simulink library "halout"  (R2024a)
settings: Solver=VariableStepAuto  StartTime=0.0  StopTime=10.0  RelTol=1e-3
undefined symbols (not defined in the file): KHAL_CAN3TxReq_flg, KHAL_CAN_MCU_R1TxReq_flg, TRUE
libraries: FVT_lib x20, simulink x1
settings Model: Creator=13168  LastModifiedBy=FVT22063
settings SolverCC: AlgebraicLoopSolver=TrustRegion
settings DataIOCC: SaveFormat=Array  SignalLoggingSaveFormat=ModelDataLogs  ReturnWorkspaceOutputs=off
settings OptimizationCC: BlockReduction=off  BooleanDataType=off
settings DebuggingCC: SaveWithParameterizedLinksMsg=none  UnderspecifiedInitializationDetection=Classic  MergeDetectMultiDrivingBlocksExec=none  SignalResolutionControl=TryResolveAllWithWarning  UnconnectedInputMsg=warning  UnconnectedOutputMsg=warning  UnconnectedLineMsg=warning
settings HardwareCC: TargetUnknown=on
settings ModelReferenceCC: EnableRefExpFcnMdlSchedulingChecks=on  PropagateSignalLabelsOutOfModel=off
settings RTWCC: GPUComputeCapability=3.5  DLArmComputeVersion=19.05
settings ConfigComp: CovMetricSettings=dw  CovSaveCumulativeToWorkspaceVar=on  CovSaveSingleToWorkspaceVar=on

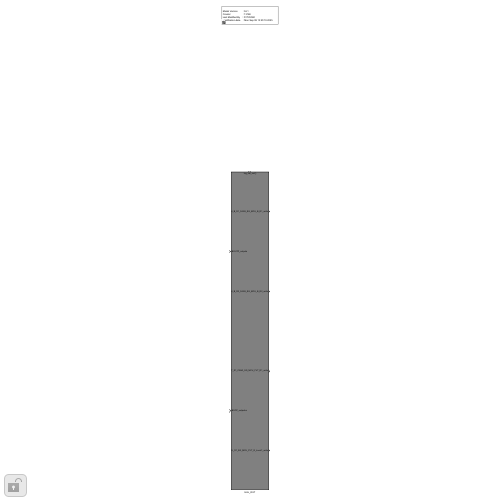
[thumbnail: Simulink's stored preview of the top-level diagram]
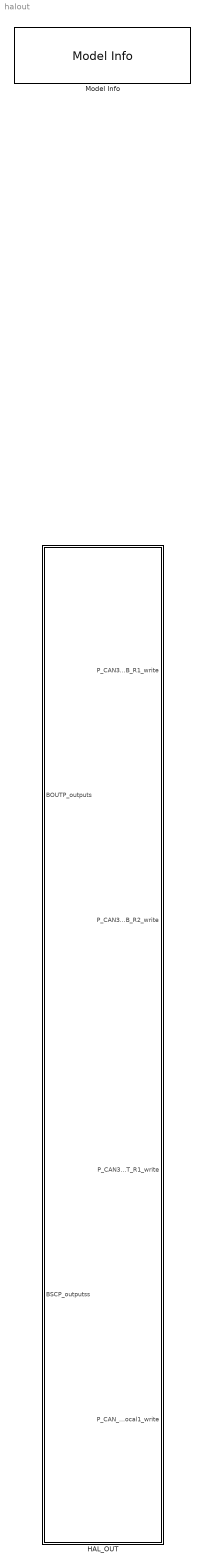
== system halout ==
  HAL_OUT : Subsystem
      settings: RTWSystemCode=Nonreusable function  RTWFcnNameOpts=Use subsystem name  RTWFileNameOpts=Use subsystem name
  Model Info : simulink/Model-Wide Utilities/Model Info  Frame=on  DisplayStringWithTags=|  HorizontalTextAlignment=Left  LeftAlignmentValue=0.02
      | Model Version        : %<ModelVersion>
      | Creator                   : %<Creator>
      | Last Modified By    : %<LastModifiedBy>
      | Modification date    : %<LastModificationDate>

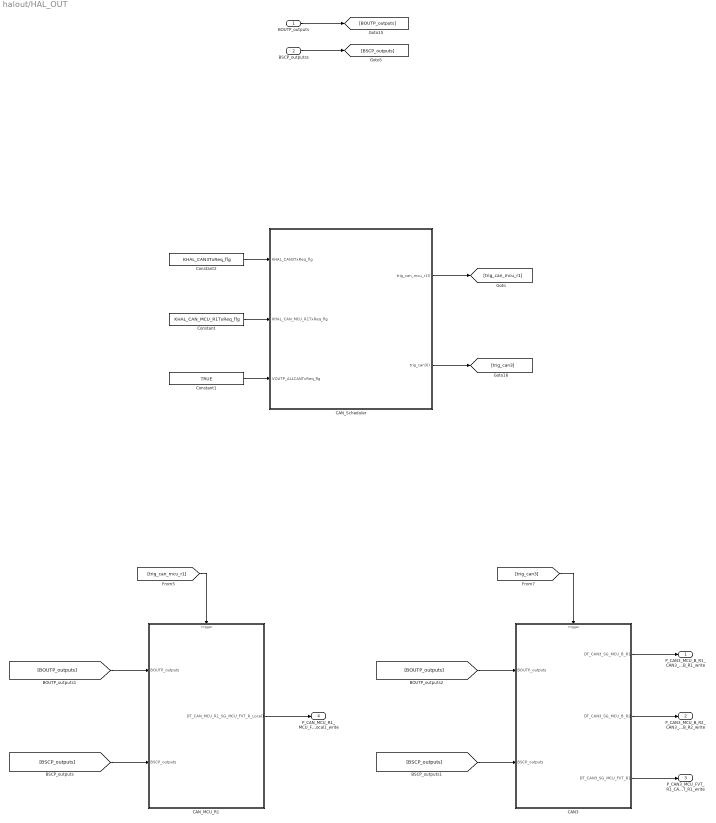
== system halout/HAL_OUT ==
  BOUTP_outputs : Inport  OutDataTypeStr=Bus: BOUTP_outputs
  BSCP_outputss : Inport  Port=2  OutDataTypeStr=Bus:BSCP_outputs
  CAN3 : Subsystem  TreatAsAtomicUnit=on
  CAN_MCU_R1 : Subsystem  TreatAsAtomicUnit=on
  CAN_Scheduler : Stateflow chart  TreatAsAtomicUnit=on
      settings: PortSchema="{\"entries\":[{\"content\":{\"sides\":[{\"content\":{\"connectorIds\":[\"In1\",\"In3\",\"In2\"]},\"type\":\"ConnectorPlacement.EquallySpacedRectSide\",\"uuid\":\"eca17bd2-3cd0-45cb-a786-10f6e0edb75c\"},{\"content\":{\"connectorIds\":[\"Out1\",\"Out2\"],\"side\":\"RIGHT\"},\"type\":\"ConnectorPlacement.EquallySpacedRectSide\",\"uuid\":\"6e53f934-0f1a-471e-8062-0040e0751220\"},{\"content\":{\"side\":\"TOP\"},\"type\":\"ConnectorPlacement.EquallySpacedRectSide\",\"uuid\":\"8d6d34ea-7fb8-416e-91ba-08d9a797d464\"}]},\"type\":\"ConnectorPlacement.EquallySpacedConnector\",\"uuid\":\"7b75ce71-1842-4580-bcde-4badbb5525c1\"}],\"packageUris\":[\"http://schema.mathworks.com/mf0/Connector/R2020b\"],\"version\":\"1.0\"}"
  Constant : Constant  Value=KHAL_CAN_MCU_R1TxReq_flg
  Constant1 : Constant  Value=TRUE  OutDataTypeStr=boolean
  Constant2 : Constant  Value=KHAL_CAN3TxReq_flg
  P_CAN3_MCU_B_R1_CAN3_SG_MCU_B_R1_write : Outport  OutDataTypeStr=Bus: DT_CAN3_SG_MCU_B_R1
  P_CAN3_MCU_B_R2_CAN3_SG_MCU_B_R2_write : Outport  Port=2  OutDataTypeStr=Bus: DT_CAN3_SG_MCU_B_R2
  P_CAN3_MCU_FVT_R1_CAN3_SG_MCU_FVT_R1_write : Outport  Port=3  OutDataTypeStr=Bus: DT_CAN3_SG_MCU_FVT_R1
  P_CAN_MCU_R1_MCU_FVT_R_Local1_CAN_MCU_R1_SG_MCU_FVT_R_Local1_write : Outport  Port=4  OutDataTypeStr=Bus: DT_CAN_MCU_R1_SG_MCU_FVT_R_Local1
  wires:
  BSCP_outputss/1 -> [BSCP_outputs]
  BOUTP_outputs/1 -> [BOUTP_outputs]
  Constant/1 -> CAN_Scheduler/3(KHAL_CAN_MCU_R1TxReq_flg)
  Constant2/1 -> CAN_Scheduler/1(KHAL_CAN3TxReq_flg)
  Constant1/1 -> CAN_Scheduler/2(VOUTP_ALLCANTxReq_flg)
  CAN_Scheduler/2(trig_can3()) -> [trig_can3]
  CAN_Scheduler/1(trig_can_mcu_r1()) -> [trig_can_mcu_r1]
  [trig_can3] -> CAN3/Trigger
  [trig_can_mcu_r1] -> CAN_MCU_R1/Trigger
  [BOUTP_outputs] -> CAN3/1(BOUTP_outputs)
  CAN3/2(DT_CAN3_SG_MCU_B_R2) -> P_CAN3_MCU_B_R2_CAN3_SG_MCU_B_R2_write/1
  [BSCP_outputs] -> CAN_MCU_R1/2(BSCP_outputs)
  [BOUTP_outputs] -> CAN_MCU_R1/1(BOUTP_outputs)
  CAN3/1(DT_CAN3_SG_MCU_B_R1) -> P_CAN3_MCU_B_R1_CAN3_SG_MCU_B_R1_write/1
  CAN_MCU_R1/1(DT_CAN_MCU_R1_SG_MCU_FVT_R_Local1) -> P_CAN_MCU_R1_MCU_FVT_R_Local1_CAN_MCU_R1_SG_MCU_FVT_R_Local1_write/1
  [BSCP_outputs] -> CAN3/2(BSCP_outputs)
  CAN3/3(DT_CAN3_SG_MCU_FVT_R1) -> P_CAN3_MCU_FVT_R1_CAN3_SG_MCU_FVT_R1_write/1

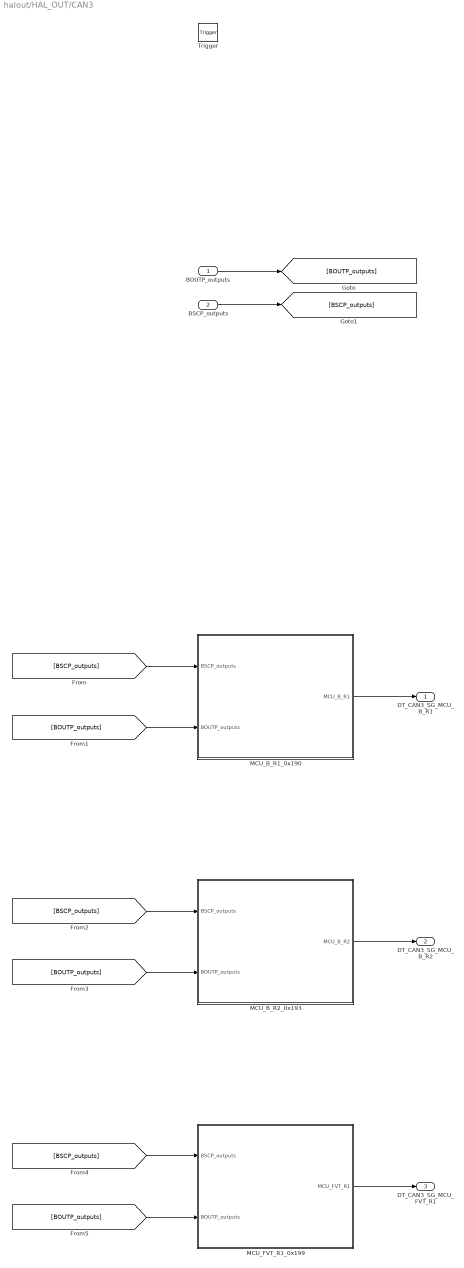
== system halout/HAL_OUT/CAN3 ==
  BOUTP_outputs : Inport  OutDataTypeStr=Bus: BOUTP_outputs
  BSCP_outputs : Inport  Port=2  OutDataTypeStr=Bus: BSCP_outputs
  Trigger : TriggerPort  TriggerType=function-call  VariantControl=(inherit)
  MCU_B_R1_0x190 : Subsystem
  MCU_B_R2_0x193 : Subsystem
  MCU_FVT_R1_0x199 : Subsystem
  DT_CAN3_SG_MCU_B_R1 : Outport  OutDataTypeStr=Bus: DT_CAN3_SG_MCU_B_R1
  DT_CAN3_SG_MCU_B_R2 : Outport  Port=2  OutDataTypeStr=Bus: DT_CAN3_SG_MCU_B_R2
  DT_CAN3_SG_MCU_FVT_R1 : Outport  Port=3  OutDataTypeStr=Bus: DT_CAN3_SG_MCU_FVT_R1
  wires:
  BOUTP_outputs/1 -> [BOUTP_outputs]
  BSCP_outputs/1 -> [BSCP_outputs]
  [BSCP_outputs] -> MCU_B_R1_0x190/1(BSCP_outputs)
  [BOUTP_outputs] -> MCU_B_R1_0x190/2(BOUTP_outputs)
  MCU_B_R1_0x190/1(MCU_B_R1) -> DT_CAN3_SG_MCU_B_R1/1
  [BSCP_outputs] -> MCU_B_R2_0x193/1(BSCP_outputs)
  [BOUTP_outputs] -> MCU_B_R2_0x193/2(BOUTP_outputs)
  MCU_B_R2_0x193/1(MCU_B_R2) -> DT_CAN3_SG_MCU_B_R2/1
  [BSCP_outputs] -> MCU_FVT_R1_0x199/1(BSCP_outputs)
  [BOUTP_outputs] -> MCU_FVT_R1_0x199/2(BOUTP_outputs)
  MCU_FVT_R1_0x199/1(MCU_FVT_R1) -> DT_CAN3_SG_MCU_FVT_R1/1

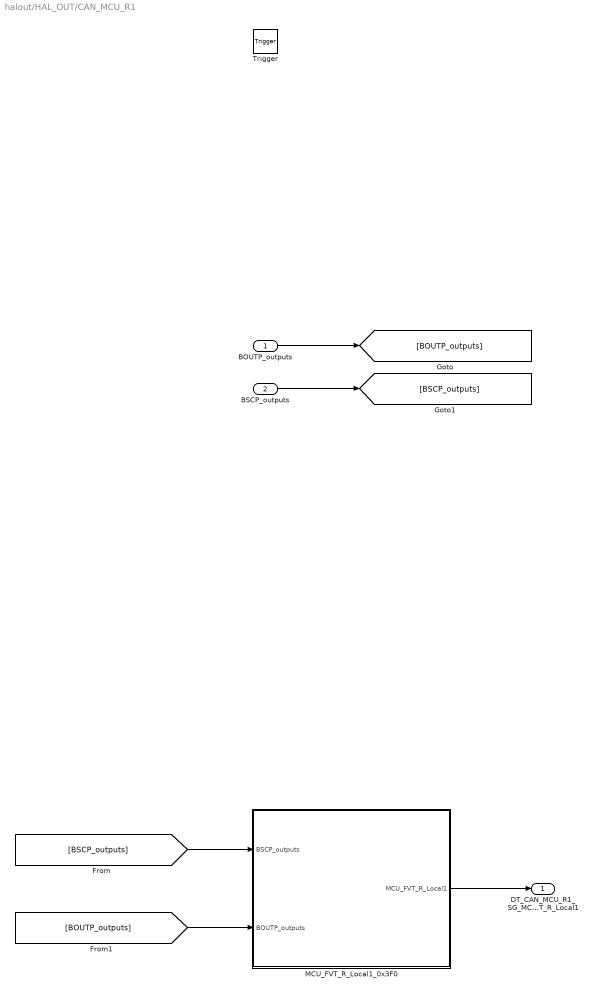
== system halout/HAL_OUT/CAN_MCU_R1 ==
  BOUTP_outputs : Inport  OutDataTypeStr=Bus: BOUTP_outputs
  BSCP_outputs : Inport  Port=2  OutDataTypeStr=Bus: BSCP_outputs
  Trigger : TriggerPort  TriggerType=function-call  VariantControl=(inherit)
  MCU_FVT_R_Local1_0x3F0 : Subsystem
  DT_CAN_MCU_R1_SG_MCU_FVT_R_Local1 : Outport  OutDataTypeStr=Bus: DT_CAN_MCU_R1_SG_MCU_FVT_R_Local1
  wires:
  BOUTP_outputs/1 -> [BOUTP_outputs]
  BSCP_outputs/1 -> [BSCP_outputs]
  [BSCP_outputs] -> MCU_FVT_R_Local1_0x3F0/1(BSCP_outputs)
  [BOUTP_outputs] -> MCU_FVT_R_Local1_0x3F0/2(BOUTP_outputs)
  MCU_FVT_R_Local1_0x3F0/1(MCU_FVT_R_Local1) -> DT_CAN_MCU_R1_SG_MCU_FVT_R_Local1/1

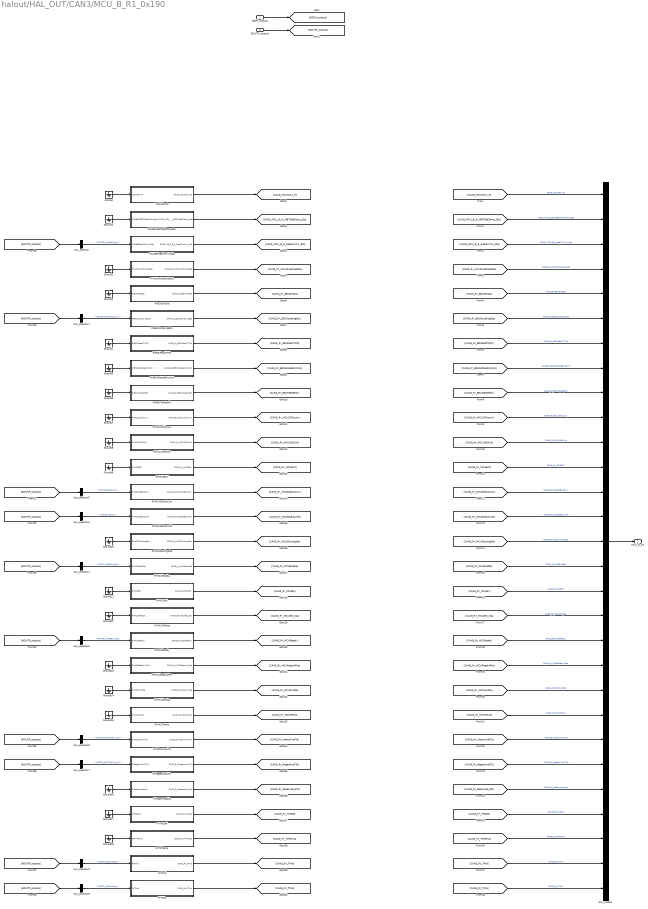
== system halout/HAL_OUT/CAN3/MCU_B_R1_0x190 ==
  BSCP_outputs : Inport  OutDataTypeStr=Bus: BSCP_outputs
  BOUTP_outputs : Inport  Port=2  OutDataTypeStr=Bus: BOUTP_outputs
  Ground{,1..18} (19 alike) : Ground
  MCUBRIGBTDdeTempSta : Subsystem
  MCUBRRealPwrKwSta : Subsystem
  MCUWarnR : Subsystem
  RrActvDmpDisabSta : Subsystem
  RrEDUDrtSta : Subsystem
  RrEDUOpratingSta : Subsystem
  RrEDURealTMTq : Subsystem
  RrEDURotateDirction : Subsystem
  RrEDUTqReqFbk : Subsystem
  RrMCU1Chksum : Subsystem
  RrMCU1RolCnt : Subsystem
  RrMCUBAT : Subsystem
  RrMCUDCBusCurr : Subsystem
  RrMCUDCBusVolt : Subsystem
  RrMCUDischrgSta : Subsystem
  RrMCUEnaSta : Subsystem
  RrMCUErr : Subsystem
  RrMCUIGNsta : Subsystem
  RrMCUReady : Subsystem
  RrMCUReady4Pre : Subsystem
  RrMCUSysSta : Subsystem
  RrMCUTemp : Subsystem
  RrMotorAvailTq : Subsystem
  RrRegenAvailTq : Subsystem
  RrReservedbits : Subsystem
  RrTMSpd : Subsystem
  RrTMTemp : Subsystem
  RrTMid : Subsystem
  RrTMiq : Subsystem
  bus_creator : BusCreator  Inputs=29  OutDataTypeStr=Bus: DT_CAN3_SG_MCU_B_R1  NonVirtualBus=on
  bus_selector : BusSelector  OutputSignals=VOUTP_PwrEleAct_W
  bus_selector1 : BusSelector  OutputSignals=VOUTP_MotMod_enum
  bus_selector2 : BusSelector  OutputSignals=VOUTP_BusCurr_A
  bus_selector3 : BusSelector  OutputSignals=VOUTP_uDC_V
  bus_selector4 : BusSelector  OutputSignals=VOUTP_MCUEna_flg
  bus_selector5 : BusSelector  OutputSignals=VOUTP_TMReady_flg
  bus_selector6 : BusSelector  OutputSignals=VOUTP_tqTMTqMax_Nm
  bus_selector7 : BusSelector  OutputSignals=VOUTP_tqTMTqMin_Nm
  bus_selector8 : BusSelector  OutputSignals=VOUTP_iDCurrAct_A
  bus_selector9 : BusSelector  OutputSignals=VOUTP_iQCurrAct_A
  MCU_B_R1 : Outport
  wires:
  BSCP_outputs/1 -> [BSCP_outputs]
  BOUTP_outputs/1 -> [BOUTP_outputs]
  [CAN3_MCUWarn_R] -> bus_creator/1  "CAN3_MCUWarn_R"
  [CAN3_MCU_B_R_IGBTDdeTemp_Sta] -> bus_creator/2  "CAN3_MCU_B_R_IGBTDdeTemp_Sta"
  [CAN3_MCU_B_R_RealPwrKw_Sta] -> bus_creator/3  "CAN3_MCU_B_R_RealPwrKw_Sta"
  [CAN3_Rr_ActvDmpDisabSta] -> bus_creator/4  "CAN3_Rr_ActvDmpDisabSta"
  [CAN3_Rr_EDUDrtSta] -> bus_creator/5  "CAN3_Rr_EDUDrtSta"
  [CAN3_Rr_EDUOpratingSta] -> bus_creator/6  "CAN3_Rr_EDUOpratingSta"
  [CAN3_Rr_EDURealTMTq] -> bus_creator/7  "CAN3_Rr_EDURealTMTq"
  [CAN3_Rr_EDURotateDirction] -> bus_creator/8  "CAN3_Rr_EDURotateDirction"
  [CAN3_Rr_EDUTqReqFbk] -> bus_creator/9  "CAN3_Rr_EDUTqReqFbk"
  [CAN3_Rr_MCU1Chksum] -> bus_creator/10  "CAN3_Rr_MCU1Chksum"
  [CAN3_Rr_MCU1RolCnt] -> bus_creator/11  "CAN3_Rr_MCU1RolCnt"
  [CAN3_Rr_MCUBAT] -> bus_creator/12  "CAN3_Rr_MCUBAT"
  [CAN3_Rr_MCUDCBusCurr] -> bus_creator/13  "CAN3_Rr_MCUDCBusCurr"
  [CAN3_Rr_MCUDCBusVolt] -> bus_creator/14  "CAN3_Rr_MCUDCBusVolt"
  [CAN3_Rr_MCUDischrgSta] -> bus_creator/15  "CAN3_Rr_MCUDischrgSta"
  [CAN3_Rr_MCUEnaSta] -> bus_creator/16  "CAN3_Rr_MCUEnaSta"
  [CAN3_Rr_MCUErr] -> bus_creator/17  "CAN3_Rr_MCUErr"
  [CAN3_Rr_MCUIGN_sta] -> bus_creator/18  "CAN3_Rr_MCUIGN_sta"
  [CAN3_Rr_MCUReady] -> bus_creator/19  "CAN3_Rr_MCUReady"
  [CAN3_Rr_MCUReady4Pre] -> bus_creator/20  "CAN3_Rr_MCUReady4Pre"
  [CAN3_Rr_MCUSysSta] -> bus_creator/21  "CAN3_Rr_MCUSysSta"
  [CAN3_Rr_MCUTemp] -> bus_creator/22  "CAN3_Rr_MCUTemp"
  [CAN3_Rr_MotorAvailTq] -> bus_creator/23  "CAN3_Rr_MotorAvailTq"
  [CAN3_Rr_RegenAvailTq] -> bus_creator/24  "CAN3_Rr_RegenAvailTq"
  [CAN3_Rr_Reserved_bits] -> bus_creator/25  "CAN3_Rr_Reserved_bits"
  [CAN3_Rr_TMSpd] -> bus_creator/26  "CAN3_Rr_TMSpd"
  [CAN3_Rr_TMTemp] -> bus_creator/27  "CAN3_Rr_TMTemp"
  [CAN3_Rr_TMid] -> bus_creator/28  "CAN3_Rr_TMid"
  [CAN3_Rr_TMiq] -> bus_creator/29  "CAN3_Rr_TMiq"
  bus_creator/1 -> MCU_B_R1/1
  MCUWarnR/1(CAN3_MCUWarn_R) -> [CAN3_MCUWarn_R]
  MCUBRIGBTDdeTempSta/1(CAN3_MCU_B_R_IGBTDdeTemp_Sta) -> [CAN3_MCU_B_R_IGBTDdeTemp_Sta]
  MCUBRRealPwrKwSta/1(CAN3_MCU_B_R_RealPwrKw_Sta) -> [CAN3_MCU_B_R_RealPwrKw_Sta]
  RrActvDmpDisabSta/1(CAN3_Rr_ActvDmpDisabSta) -> [CAN3_Rr_ActvDmpDisabSta]
  RrEDUDrtSta/1(CAN3_Rr_EDUDrtSta) -> [CAN3_Rr_EDUDrtSta]
  RrEDUOpratingSta/1(CAN3_Rr_EDUOpratingSta) -> [CAN3_Rr_EDUOpratingSta]
  RrEDURealTMTq/1(CAN3_Rr_EDURealTMTq) -> [CAN3_Rr_EDURealTMTq]
  RrEDURotateDirction/1(CAN3_Rr_EDURotateDirction) -> [CAN3_Rr_EDURotateDirction]
  RrEDUTqReqFbk/1(CAN3_Rr_EDUTqReqFbk) -> [CAN3_Rr_EDUTqReqFbk]
  RrMCU1Chksum/1(CAN3_Rr_MCU1Chksum) -> [CAN3_Rr_MCU1Chksum]
  RrMCU1RolCnt/1(CAN3_Rr_MCU1RolCnt) -> [CAN3_Rr_MCU1RolCnt]
  RrMCUBAT/1(CAN3_Rr_MCUBAT) -> [CAN3_Rr_MCUBAT]
  RrMCUDCBusCurr/1(CAN3_Rr_MCUDCBusCurr) -> [CAN3_Rr_MCUDCBusCurr]
  RrMCUDCBusVolt/1(CAN3_Rr_MCUDCBusVolt) -> [CAN3_Rr_MCUDCBusVolt]
  RrMCUDischrgSta/1(CAN3_Rr_MCUDischrgSta) -> [CAN3_Rr_MCUDischrgSta]
  RrMCUEnaSta/1(CAN3_Rr_MCUEnaSta) -> [CAN3_Rr_MCUEnaSta]
  RrMCUErr/1(CAN3_Rr_MCUErr) -> [CAN3_Rr_MCUErr]
  RrMCUIGNsta/1(CAN3_Rr_MCUIGN_sta) -> [CAN3_Rr_MCUIGN_sta]
  RrMCUReady/1(CAN3_Rr_MCUReady) -> [CAN3_Rr_MCUReady]
  RrMCUReady4Pre/1(CAN3_Rr_MCUReady4Pre) -> [CAN3_Rr_MCUReady4Pre]
  RrMCUSysSta/1(CAN3_Rr_MCUSysSta) -> [CAN3_Rr_MCUSysSta]
  RrMCUTemp/1(CAN3_Rr_MCUTemp) -> [CAN3_Rr_MCUTemp]
  RrMotorAvailTq/1(CAN3_Rr_MotorAvailTq) -> [CAN3_Rr_MotorAvailTq]
  RrRegenAvailTq/1(CAN3_Rr_RegenAvailTq) -> [CAN3_Rr_RegenAvailTq]
  RrReservedbits/1(CAN3_Rr_Reserved_bits) -> [CAN3_Rr_Reserved_bits]
  RrTMSpd/1(CAN3_Rr_TMSpd) -> [CAN3_Rr_TMSpd]
  RrTMTemp/1(CAN3_Rr_TMTemp) -> [CAN3_Rr_TMTemp]
  RrTMid/1(CAN3_Rr_TMid) -> [CAN3_Rr_TMid]
  RrTMiq/1(CAN3_Rr_TMiq) -> [CAN3_Rr_TMiq]
  Ground/1 -> MCUWarnR/1(MCUWarnR)
  Ground1/1 -> MCUBRIGBTDdeTempSta/1(MCUBRIGBTDdeTempSta)
  bus_selector/1 -> MCUBRRealPwrKwSta/1(MCUBRRealPwrKwSta)  "<VOUTP_PwrEleAct_W>"
  [BOUTP_outputs] -> bus_selector/1
  Ground2/1 -> RrActvDmpDisabSta/1(RrActvDmpDisabSta)
  Ground3/1 -> RrEDUDrtSta/1(RrEDUDrtSta)
  bus_selector1/1 -> RrEDUOpratingSta/1(RrEDUOpratingSta)  "<VOUTP_MotMod_enum>"
  [BOUTP_outputs] -> bus_selector1/1
  Ground4/1 -> RrEDURealTMTq/1(RrEDURealTMTq)
  Ground5/1 -> RrEDURotateDirction/1(RrEDURotateDirction)
  Ground6/1 -> RrEDUTqReqFbk/1(RrEDUTqReqFbk)
  Ground7/1 -> RrMCU1Chksum/1(RrMCU1Chksum)
  Ground8/1 -> RrMCU1RolCnt/1(RrMCU1RolCnt)
  Ground9/1 -> RrMCUBAT/1(RrMCUBAT)
  bus_selector2/1 -> RrMCUDCBusCurr/1(RrMCUDCBusCurr)  "<VOUTP_BusCurr_A>"
  [BOUTP_outputs] -> bus_selector2/1
  bus_selector3/1 -> RrMCUDCBusVolt/1(RrMCUDCBusVolt)  "<VOUTP_uDC_V>"
  [BOUTP_outputs] -> bus_selector3/1
  Ground10/1 -> RrMCUDischrgSta/1(RrMCUDischrgSta)
  bus_selector4/1 -> RrMCUEnaSta/1(RrMCUEnaSta)  "<VOUTP_MCUEna_flg>"
  [BOUTP_outputs] -> bus_selector4/1
  Ground11/1 -> RrMCUErr/1(RrMCUErr)
  Ground12/1 -> RrMCUIGNsta/1(RrMCUIGNsta)
  bus_selector5/1 -> RrMCUReady/1(RrMCUReady)  "<VOUTP_TMReady_flg>"
  [BOUTP_outputs] -> bus_selector5/1
  Ground13/1 -> RrMCUReady4Pre/1(RrMCUReady4Pre)
  Ground14/1 -> RrMCUSysSta/1(RrMCUSysSta)
  Ground15/1 -> RrMCUTemp/1(RrMCUTemp)
  bus_selector6/1 -> RrMotorAvailTq/1(RrMotorAvailTq)  "<VOUTP_tqTMTqMax_Nm>"
  [BOUTP_outputs] -> bus_selector6/1
  bus_selector7/1 -> RrRegenAvailTq/1(RrRegenAvailTq)  "<VOUTP_tqTMTqMin_Nm>"
  [BOUTP_outputs] -> bus_selector7/1
  Ground16/1 -> RrReservedbits/1(RrReservedbits)
  Ground17/1 -> RrTMSpd/1(RrTMSpd)
  Ground18/1 -> RrTMTemp/1(RrTMTemp)
  bus_selector8/1 -> RrTMid/1(RrTMid)  "<VOUTP_iDCurrAct_A>"
  [BOUTP_outputs] -> bus_selector8/1
  bus_selector9/1 -> RrTMiq/1(RrTMiq)  "<VOUTP_iQCurrAct_A>"
  [BOUTP_outputs] -> bus_selector9/1

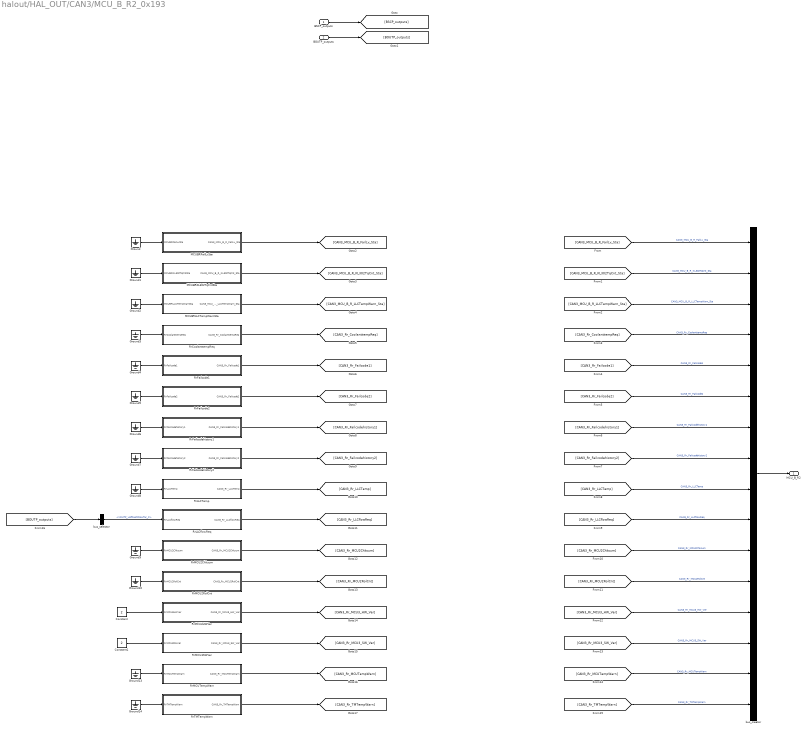
== system halout/HAL_OUT/CAN3/MCU_B_R2_0x193 ==
  BSCP_outputs : Inport  OutDataTypeStr=Bus: BSCP_outputs
  BOUTP_outputs : Inport  Port=2  OutDataTypeStr=Bus: BOUTP_outputs
  Constant : Constant  Value=2
  Constant1 : Constant  Value=2
  Ground{,1..10,13..14} (13 alike) : Ground
  MCUBRFailLvSta : Subsystem
  MCUBRKL302TqCntSta : Subsystem
  MCUBRLLCTempWarnSta : Subsystem
  RrCoolanttempReq : Subsystem
  RrFailcode1 : Subsystem
  RrFailcode2 : Subsystem
  RrFailcodehistory1 : Subsystem
  RrFailcodehistory2 : Subsystem
  RrLLCTemp : Subsystem
  RrLLCflowReq : Subsystem
  RrMCU2Chksum : Subsystem
  RrMCU2RolCnt : Subsystem
  RrMCU3HWVer : Subsystem
  RrMCU3SWVer : Subsystem
  RrMCUTempWarn : Subsystem
  RrTMTempWarn : Subsystem
  bus_creator : BusCreator  Inputs=16  OutDataTypeStr=Bus: DT_CAN3_SG_MCU_B_R2  NonVirtualBus=on
  bus_selector : BusSelector  OutputSignals=VOUTP_volfCooltFlowTar_C
  MCU_B_R2 : Outport
  wires:
  BSCP_outputs/1 -> [BSCP_outputs]
  BOUTP_outputs/1 -> [BOUTP_outputs]
  [CAN3_MCU_B_R_FailLv_Sta] -> bus_creator/1  "CAN3_MCU_B_R_FailLv_Sta"
  [CAN3_MCU_B_R_KL302TqCnt_Sta] -> bus_creator/2  "CAN3_MCU_B_R_KL302TqCnt_Sta"
  [CAN3_MCU_B_R_LLCTempWarn_Sta] -> bus_creator/3  "CAN3_MCU_B_R_LLCTempWarn_Sta"
  [CAN3_Rr_CoolanttempReq] -> bus_creator/4  "CAN3_Rr_CoolanttempReq"
  [CAN3_Rr_Failcode1] -> bus_creator/5  "CAN3_Rr_Failcode1"
  [CAN3_Rr_Failcode2] -> bus_creator/6  "CAN3_Rr_Failcode2"
  [CAN3_Rr_Failcodehistory1] -> bus_creator/7  "CAN3_Rr_Failcodehistory1"
  [CAN3_Rr_Failcodehistory2] -> bus_creator/8  "CAN3_Rr_Failcodehistory2"
  [CAN3_Rr_LLCTemp] -> bus_creator/9  "CAN3_Rr_LLCTemp"
  [CAN3_Rr_LLCflowReq] -> bus_creator/10  "CAN3_Rr_LLCflowReq"
  [CAN3_Rr_MCU2Chksum] -> bus_creator/11  "CAN3_Rr_MCU2Chksum"
  [CAN3_Rr_MCU2RolCnt] -> bus_creator/12  "CAN3_Rr_MCU2RolCnt"
  [CAN3_Rr_MCU3_HW_Ver] -> bus_creator/13  "CAN3_Rr_MCU3_HW_Ver"
  [CAN3_Rr_MCU3_SW_Ver] -> bus_creator/14  "CAN3_Rr_MCU3_SW_Ver"
  [CAN3_Rr_MCUTempWarn] -> bus_creator/15  "CAN3_Rr_MCUTempWarn"
  [CAN3_Rr_TMTempWarn] -> bus_creator/16  "CAN3_Rr_TMTempWarn"
  bus_creator/1 -> MCU_B_R2/1
  MCUBRFailLvSta/1(CAN3_MCU_B_R_FailLv_Sta) -> [CAN3_MCU_B_R_FailLv_Sta]
  MCUBRKL302TqCntSta/1(CAN3_MCU_B_R_KL302TqCnt_Sta) -> [CAN3_MCU_B_R_KL302TqCnt_Sta]
  MCUBRLLCTempWarnSta/1(CAN3_MCU_B_R_LLCTempWarn_Sta) -> [CAN3_MCU_B_R_LLCTempWarn_Sta]
  RrCoolanttempReq/1(CAN3_Rr_CoolanttempReq) -> [CAN3_Rr_CoolanttempReq]
  RrFailcode1/1(CAN3_Rr_Failcode1) -> [CAN3_Rr_Failcode1]
  RrFailcode2/1(CAN3_Rr_Failcode2) -> [CAN3_Rr_Failcode2]
  RrFailcodehistory1/1(CAN3_Rr_Failcodehistory1) -> [CAN3_Rr_Failcodehistory1]
  RrFailcodehistory2/1(CAN3_Rr_Failcodehistory2) -> [CAN3_Rr_Failcodehistory2]
  RrLLCTemp/1(CAN3_Rr_LLCTemp) -> [CAN3_Rr_LLCTemp]
  RrLLCflowReq/1(CAN3_Rr_LLCflowReq) -> [CAN3_Rr_LLCflowReq]
  RrMCU2Chksum/1(CAN3_Rr_MCU2Chksum) -> [CAN3_Rr_MCU2Chksum]
  RrMCU2RolCnt/1(CAN3_Rr_MCU2RolCnt) -> [CAN3_Rr_MCU2RolCnt]
  RrMCU3HWVer/1(CAN3_Rr_MCU3_HW_Ver) -> [CAN3_Rr_MCU3_HW_Ver]
  RrMCU3SWVer/1(CAN3_Rr_MCU3_SW_Ver) -> [CAN3_Rr_MCU3_SW_Ver]
  RrMCUTempWarn/1(CAN3_Rr_MCUTempWarn) -> [CAN3_Rr_MCUTempWarn]
  RrTMTempWarn/1(CAN3_Rr_TMTempWarn) -> [CAN3_Rr_TMTempWarn]
  Ground/1 -> MCUBRFailLvSta/1(MCUBRFailLvSta)
  Ground1/1 -> MCUBRKL302TqCntSta/1(MCUBRKL302TqCntSta)
  Ground2/1 -> MCUBRLLCTempWarnSta/1(MCUBRLLCTempWarnSta)
  Ground3/1 -> RrCoolanttempReq/1(RrCoolanttempReq)
  Ground4/1 -> RrFailcode1/1(RrFailcode1)
  Ground5/1 -> RrFailcode2/1(RrFailcode2)
  Ground6/1 -> RrFailcodehistory1/1(RrFailcodehistory1)
  Ground7/1 -> RrFailcodehistory2/1(RrFailcodehistory2)
  Ground8/1 -> RrLLCTemp/1(RrLLCTemp)
  bus_selector/1 -> RrLLCflowReq/1(RrLLCflowReq)  "<VOUTP_volfCooltFlowTar_C>"
  [BOUTP_outputs] -> bus_selector/1
  Ground9/1 -> RrMCU2Chksum/1(RrMCU2Chksum)
  Ground10/1 -> RrMCU2RolCnt/1(RrMCU2RolCnt)
  Constant/1 -> RrMCU3HWVer/1(RrMCU3HWVer)
  Constant1/1 -> RrMCU3SWVer/1(RrMCU3SWVer)
  Ground13/1 -> RrMCUTempWarn/1(RrMCUTempWarn)
  Ground14/1 -> RrTMTempWarn/1(RrTMTempWarn)

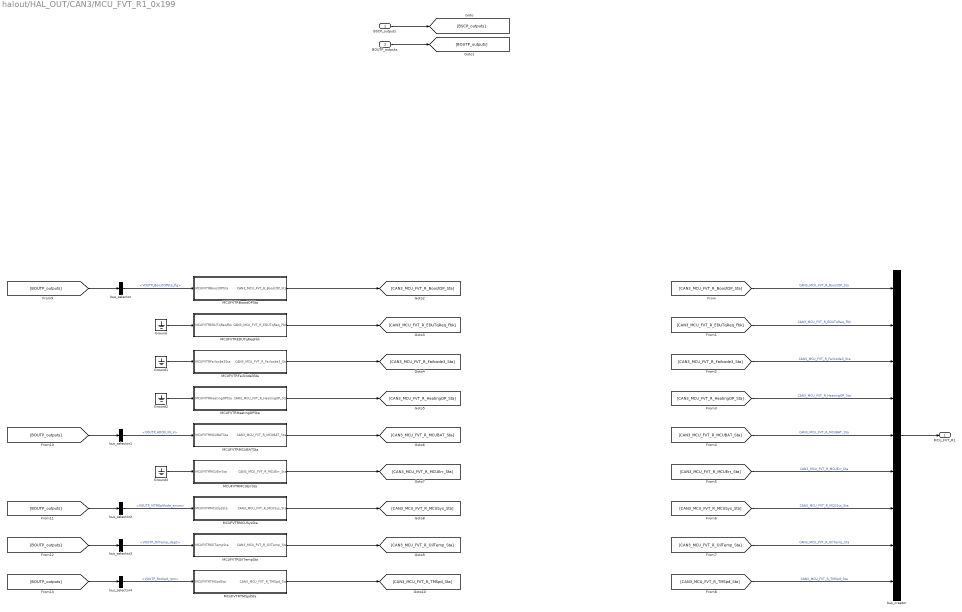
== system halout/HAL_OUT/CAN3/MCU_FVT_R1_0x199 ==
  BSCP_outputs : Inport  OutDataTypeStr=Bus: BSCP_outputs
  BOUTP_outputs : Inport  Port=2  OutDataTypeStr=Bus: BOUTP_outputs
  Ground{,1..3} (4 alike) : Ground
  MCUFVTRBoostOPSta : Subsystem
  MCUFVTREDUTqReqFbk : Subsystem
  MCUFVTRFailcode3Sta : Subsystem
  MCUFVTRHeatingOPSta : Subsystem
  MCUFVTRMCUBATSta : Subsystem
  MCUFVTRMCUErrSta : Subsystem
  MCUFVTRMCUSysSta : Subsystem
  MCUFVTROilTempSta : Subsystem
  MCUFVTRTMSpdSta : Subsystem
  bus_creator : BusCreator  Inputs=9  OutDataTypeStr=Bus: DT_CAN3_SG_MCU_FVT_R1  NonVirtualBus=on
  bus_selector : BusSelector  OutputSignals=VOUTP_BoostOPSta_flg
  bus_selector1 : BusSelector  OutputSignals=VOUTP_ADCKL30_V
  bus_selector2 : BusSelector  OutputSignals=VOUTP_IVTROpMode_enum
  bus_selector3 : BusSelector  OutputSignals=VOUTP_OilTemp_degC
  bus_selector4 : BusSelector  OutputSignals=VOUTP_RotSpd_rpm
  MCU_FVT_R1 : Outport
  wires:
  BSCP_outputs/1 -> [BSCP_outputs]
  BOUTP_outputs/1 -> [BOUTP_outputs]
  [CAN3_MCU_FVT_R_BoostOP_Sta] -> bus_creator/1  "CAN3_MCU_FVT_R_BoostOP_Sta"
  [CAN3_MCU_FVT_R_EDUTqReq_Fbk] -> bus_creator/2  "CAN3_MCU_FVT_R_EDUTqReq_Fbk"
  [CAN3_MCU_FVT_R_Failcode3_Sta] -> bus_creator/3  "CAN3_MCU_FVT_R_Failcode3_Sta"
  [CAN3_MCU_FVT_R_HeatingOP_Sta] -> bus_creator/4  "CAN3_MCU_FVT_R_HeatingOP_Sta"
  [CAN3_MCU_FVT_R_MCUBAT_Sta] -> bus_creator/5  "CAN3_MCU_FVT_R_MCUBAT_Sta"
  [CAN3_MCU_FVT_R_MCUErr_Sta] -> bus_creator/6  "CAN3_MCU_FVT_R_MCUErr_Sta"
  [CAN3_MCU_FVT_R_MCUSys_Sta] -> bus_creator/7  "CAN3_MCU_FVT_R_MCUSys_Sta"
  [CAN3_MCU_FVT_R_OilTemp_Sta] -> bus_creator/8  "CAN3_MCU_FVT_R_OilTemp_Sta"
  [CAN3_MCU_FVT_R_TMSpd_Sta] -> bus_creator/9  "CAN3_MCU_FVT_R_TMSpd_Sta"
  bus_creator/1 -> MCU_FVT_R1/1
  MCUFVTRBoostOPSta/1(CAN3_MCU_FVT_R_BoostOP_Sta) -> [CAN3_MCU_FVT_R_BoostOP_Sta]
  MCUFVTREDUTqReqFbk/1(CAN3_MCU_FVT_R_EDUTqReq_Fbk) -> [CAN3_MCU_FVT_R_EDUTqReq_Fbk]
  MCUFVTRFailcode3Sta/1(CAN3_MCU_FVT_R_Failcode3_Sta) -> [CAN3_MCU_FVT_R_Failcode3_Sta]
  MCUFVTRHeatingOPSta/1(CAN3_MCU_FVT_R_HeatingOP_Sta) -> [CAN3_MCU_FVT_R_HeatingOP_Sta]
  MCUFVTRMCUBATSta/1(CAN3_MCU_FVT_R_MCUBAT_Sta) -> [CAN3_MCU_FVT_R_MCUBAT_Sta]
  MCUFVTRMCUErrSta/1(CAN3_MCU_FVT_R_MCUErr_Sta) -> [CAN3_MCU_FVT_R_MCUErr_Sta]
  MCUFVTRMCUSysSta/1(CAN3_MCU_FVT_R_MCUSys_Sta) -> [CAN3_MCU_FVT_R_MCUSys_Sta]
  MCUFVTROilTempSta/1(CAN3_MCU_FVT_R_OilTemp_Sta) -> [CAN3_MCU_FVT_R_OilTemp_Sta]
  MCUFVTRTMSpdSta/1(CAN3_MCU_FVT_R_TMSpd_Sta) -> [CAN3_MCU_FVT_R_TMSpd_Sta]
  bus_selector/1 -> MCUFVTRBoostOPSta/1(MCUFVTRBoostOPSta)  "<VOUTP_BoostOPSta_flg>"
  [BOUTP_outputs] -> bus_selector/1
  Ground/1 -> MCUFVTREDUTqReqFbk/1(MCUFVTREDUTqReqFbk)
  Ground1/1 -> MCUFVTRFailcode3Sta/1(MCUFVTRFailcode3Sta)
  Ground2/1 -> MCUFVTRHeatingOPSta/1(MCUFVTRHeatingOPSta)
  bus_selector1/1 -> MCUFVTRMCUBATSta/1(MCUFVTRMCUBATSta)  "<VOUTP_ADCKL30_V>"
  [BOUTP_outputs] -> bus_selector1/1
  Ground3/1 -> MCUFVTRMCUErrSta/1(MCUFVTRMCUErrSta)
  bus_selector2/1 -> MCUFVTRMCUSysSta/1(MCUFVTRMCUSysSta)  "<VOUTP_IVTROpMode_enum>"
  [BOUTP_outputs] -> bus_selector2/1
  bus_selector3/1 -> MCUFVTROilTempSta/1(MCUFVTROilTempSta)  "<VOUTP_OilTemp_degC>"
  [BOUTP_outputs] -> bus_selector3/1
  bus_selector4/1 -> MCUFVTRTMSpdSta/1(MCUFVTRTMSpdSta)  "<VOUTP_RotSpd_rpm>"
  [BOUTP_outputs] -> bus_selector4/1

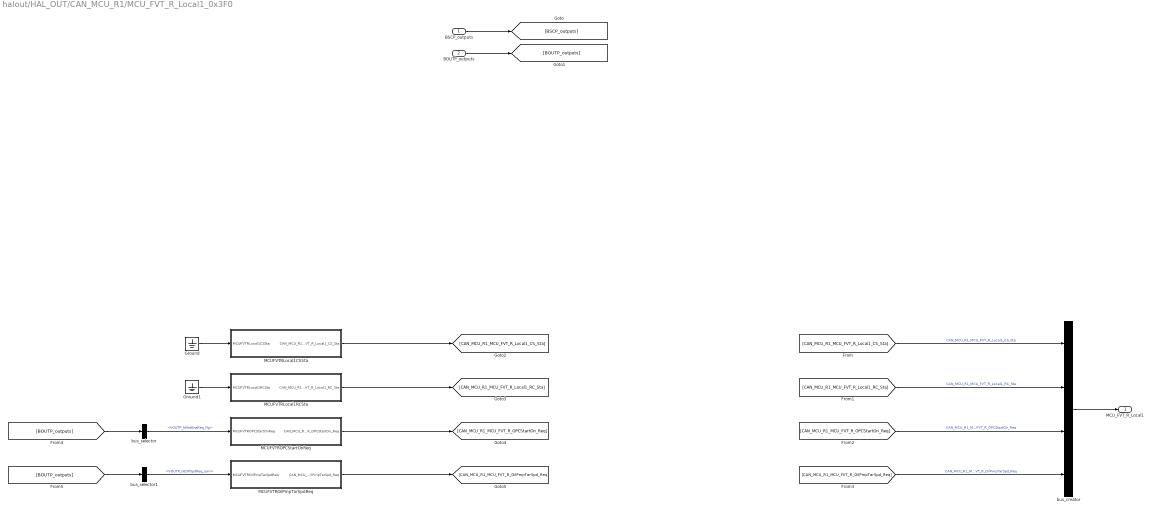
== system halout/HAL_OUT/CAN_MCU_R1/MCU_FVT_R_Local1_0x3F0 ==
  BSCP_outputs : Inport  OutDataTypeStr=Bus: BSCP_outputs
  BOUTP_outputs : Inport  Port=2  OutDataTypeStr=Bus: BOUTP_outputs
  Ground : Ground
  Ground1 : Ground
  MCUFVTRLocal1CSSta : Subsystem
  MCUFVTRLocal1RCSta : Subsystem
  MCUFVTROPCStartOnReq : Subsystem
  MCUFVTROilPmpTarSpdReq : Subsystem
  bus_creator : BusCreator  Inputs=4  OutDataTypeStr=Bus: DT_CAN_MCU_R1_SG_MCU_FVT_R_Local1  NonVirtualBus=on
  bus_selector : BusSelector  OutputSignals=VOUTP_bMotEnaReq_flg
  bus_selector1 : BusSelector  OutputSignals=VOUTP_nEOPSpdReq_rpm
  MCU_FVT_R_Local1 : Outport
  wires:
  BSCP_outputs/1 -> [BSCP_outputs]
  BOUTP_outputs/1 -> [BOUTP_outputs]
  [CAN_MCU_R1_MCU_FVT_R_Local1_CS_Sta] -> bus_creator/1  "CAN_MCU_R1_MCU_FVT_R_Local1_CS_Sta"
  [CAN_MCU_R1_MCU_FVT_R_Local1_RC_Sta] -> bus_creator/2  "CAN_MCU_R1_MCU_FVT_R_Local1_RC_Sta"
  [CAN_MCU_R1_MCU_FVT_R_OPCStartOn_Req] -> bus_creator/3  "CAN_MCU_R1_MCU_FVT_R_OPCStartOn_Req"
  [CAN_MCU_R1_MCU_FVT_R_OilPmpTarSpd_Req] -> bus_creator/4  "CAN_MCU_R1_MCU_FVT_R_OilPmpTarSpd_Req"
  bus_creator/1 -> MCU_FVT_R_Local1/1
  MCUFVTRLocal1CSSta/1(CAN_MCU_R1_MCU_FVT_R_Local1_CS_Sta) -> [CAN_MCU_R1_MCU_FVT_R_Local1_CS_Sta]
  MCUFVTRLocal1RCSta/1(CAN_MCU_R1_MCU_FVT_R_Local1_RC_Sta) -> [CAN_MCU_R1_MCU_FVT_R_Local1_RC_Sta]
  MCUFVTROPCStartOnReq/1(CAN_MCU_R1_MCU_FVT_R_OPCStartOn_Req) -> [CAN_MCU_R1_MCU_FVT_R_OPCStartOn_Req]
  MCUFVTROilPmpTarSpdReq/1(CAN_MCU_R1_MCU_FVT_R_OilPmpTarSpd_Req) -> [CAN_MCU_R1_MCU_FVT_R_OilPmpTarSpd_Req]
  Ground/1 -> MCUFVTRLocal1CSSta/1(MCUFVTRLocal1CSSta)
  Ground1/1 -> MCUFVTRLocal1RCSta/1(MCUFVTRLocal1RCSta)
  bus_selector/1 -> MCUFVTROPCStartOnReq/1(MCUFVTROPCStartOnReq)  "<VOUTP_bMotEnaReq_flg>"
  [BOUTP_outputs] -> bus_selector/1
  bus_selector1/1 -> MCUFVTROilPmpTarSpdReq/1(MCUFVTROilPmpTarSpdReq)  "<VOUTP_nEOPSpdReq_rpm>"
  [BOUTP_outputs] -> bus_selector1/1

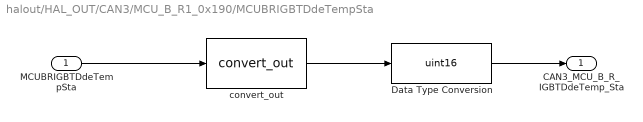
== system halout/HAL_OUT/CAN3/MCU_B_R1_0x190/MCUBRIGBTDdeTempSta ==
  MCUBRIGBTDdeTempSta : Inport
  Data Type Conversion : DataTypeConversion  OutDataTypeStr=uint16  RndMeth=Round  SaturateOnIntegerOverflow=off
  convert_out : FVT_lib/hal/convert_out  gain=1  offset=-40
  CAN3_MCU_B_R_IGBTDdeTemp_Sta : Outport
  wires:
  Data Type Conversion/1 -> CAN3_MCU_B_R_IGBTDdeTemp_Sta/1
  convert_out/1 -> Data Type Conversion/1
  MCUBRIGBTDdeTempSta/1 -> convert_out/1

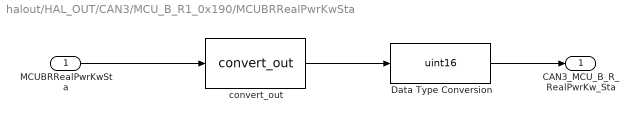
== system halout/HAL_OUT/CAN3/MCU_B_R1_0x190/MCUBRRealPwrKwSta ==
  MCUBRRealPwrKwSta : Inport
  Data Type Conversion : DataTypeConversion  OutDataTypeStr=uint16  RndMeth=Round  SaturateOnIntegerOverflow=off
  convert_out : FVT_lib/hal/convert_out  gain=0.1  offset=-530
  CAN3_MCU_B_R_RealPwrKw_Sta : Outport
  wires:
  Data Type Conversion/1 -> CAN3_MCU_B_R_RealPwrKw_Sta/1
  convert_out/1 -> Data Type Conversion/1
  MCUBRRealPwrKwSta/1 -> convert_out/1

== system halout/HAL_OUT/CAN3/MCU_B_R1_0x190/MCUWarnR ==
  MCUWarnR : Inport
  Data Type Conversion : DataTypeConversion  OutDataTypeStr=uint8  RndMeth=Round  SaturateOnIntegerOverflow=off
  CAN3_MCUWarn_R : Outport
  wires:
  Data Type Conversion/1 -> CAN3_MCUWarn_R/1
  MCUWarnR/1 -> Data Type Conversion/1

== system halout/HAL_OUT/CAN3/MCU_B_R1_0x190/RrActvDmpDisabSta ==
  RrActvDmpDisabSta : Inport
  Data Type Conversion : DataTypeConversion  OutDataTypeStr=uint8  RndMeth=Round  SaturateOnIntegerOverflow=off
  CAN3_Rr_ActvDmpDisabSta : Outport
  wires:
  Data Type Conversion/1 -> CAN3_Rr_ActvDmpDisabSta/1
  RrActvDmpDisabSta/1 -> Data Type Conversion/1

== system halout/HAL_OUT/CAN3/MCU_B_R1_0x190/RrEDUDrtSta ==
  RrEDUDrtSta : Inport
  Data Type Conversion : DataTypeConversion  OutDataTypeStr=uint8  RndMeth=Round  SaturateOnIntegerOverflow=off
  CAN3_Rr_EDUDrtSta : Outport
  wires:
  Data Type Conversion/1 -> CAN3_Rr_EDUDrtSta/1
  RrEDUDrtSta/1 -> Data Type Conversion/1

== system halout/HAL_OUT/CAN3/MCU_B_R1_0x190/RrEDUOpratingSta ==
  RrEDUOpratingSta : Inport
  Data Type Conversion : DataTypeConversion  OutDataTypeStr=uint8  RndMeth=Round  SaturateOnIntegerOverflow=off
  CAN3_Rr_EDUOpratingSta : Outport
  wires:
  Data Type Conversion/1 -> CAN3_Rr_EDUOpratingSta/1
  RrEDUOpratingSta/1 -> Data Type Conversion/1

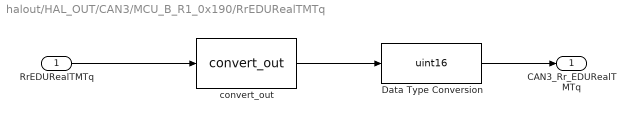
== system halout/HAL_OUT/CAN3/MCU_B_R1_0x190/RrEDURealTMTq ==
  RrEDURealTMTq : Inport
  Data Type Conversion : DataTypeConversion  OutDataTypeStr=uint16  RndMeth=Round  SaturateOnIntegerOverflow=off
  convert_out : FVT_lib/hal/convert_out  gain=0.1  offset=-1022
  CAN3_Rr_EDURealTMTq : Outport
  wires:
  Data Type Conversion/1 -> CAN3_Rr_EDURealTMTq/1
  convert_out/1 -> Data Type Conversion/1
  RrEDURealTMTq/1 -> convert_out/1

== system halout/HAL_OUT/CAN3/MCU_B_R1_0x190/RrEDURotateDirction ==
  RrEDURotateDirction : Inport
  Data Type Conversion : DataTypeConversion  OutDataTypeStr=uint8  RndMeth=Round  SaturateOnIntegerOverflow=off
  CAN3_Rr_EDURotateDirction : Outport
  wires:
  Data Type Conversion/1 -> CAN3_Rr_EDURotateDirction/1
  RrEDURotateDirction/1 -> Data Type Conversion/1

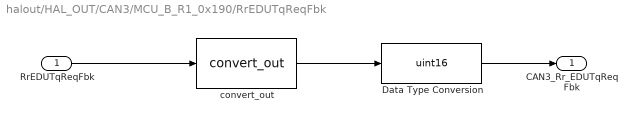
== system halout/HAL_OUT/CAN3/MCU_B_R1_0x190/RrEDUTqReqFbk ==
  RrEDUTqReqFbk : Inport
  Data Type Conversion : DataTypeConversion  OutDataTypeStr=uint16  RndMeth=Round  SaturateOnIntegerOverflow=off
  convert_out : FVT_lib/hal/convert_out  gain=1  offset=-1022
  CAN3_Rr_EDUTqReqFbk : Outport
  wires:
  Data Type Conversion/1 -> CAN3_Rr_EDUTqReqFbk/1
  convert_out/1 -> Data Type Conversion/1
  RrEDUTqReqFbk/1 -> convert_out/1

== system halout/HAL_OUT/CAN3/MCU_B_R1_0x190/RrMCU1Chksum ==
  RrMCU1Chksum : Inport
  Data Type Conversion : DataTypeConversion  OutDataTypeStr=uint8  RndMeth=Round  SaturateOnIntegerOverflow=off
  CAN3_Rr_MCU1Chksum : Outport
  wires:
  Data Type Conversion/1 -> CAN3_Rr_MCU1Chksum/1
  RrMCU1Chksum/1 -> Data Type Conversion/1

== system halout/HAL_OUT/CAN3/MCU_B_R1_0x190/RrMCU1RolCnt ==
  RrMCU1RolCnt : Inport
  Data Type Conversion : DataTypeConversion  OutDataTypeStr=uint8  RndMeth=Round  SaturateOnIntegerOverflow=off
  CAN3_Rr_MCU1RolCnt : Outport
  wires:
  Data Type Conversion/1 -> CAN3_Rr_MCU1RolCnt/1
  RrMCU1RolCnt/1 -> Data Type Conversion/1

== system halout/HAL_OUT/CAN3/MCU_B_R1_0x190/RrMCUBAT ==
  RrMCUBAT : Inport
  Data Type Conversion : DataTypeConversion  OutDataTypeStr=uint8  RndMeth=Round  SaturateOnIntegerOverflow=off
  convert_out : FVT_lib/hal/convert_out  gain=0.1  offset=0
  CAN3_Rr_MCUBAT : Outport
  wires:
  Data Type Conversion/1 -> CAN3_Rr_MCUBAT/1
  convert_out/1 -> Data Type Conversion/1
  RrMCUBAT/1 -> convert_out/1

== system halout/HAL_OUT/CAN3/MCU_B_R1_0x190/RrMCUDCBusCurr ==
  RrMCUDCBusCurr : Inport
  Data Type Conversion : DataTypeConversion  OutDataTypeStr=uint16  RndMeth=Round  SaturateOnIntegerOverflow=off
  convert_out : FVT_lib/hal/convert_out  gain=0.1  offset=-1500
  CAN3_Rr_MCUDCBusCurr : Outport
  wires:
  Data Type Conversion/1 -> CAN3_Rr_MCUDCBusCurr/1
  convert_out/1 -> Data Type Conversion/1
  RrMCUDCBusCurr/1 -> convert_out/1

== system halout/HAL_OUT/CAN3/MCU_B_R1_0x190/RrMCUDCBusVolt ==
  RrMCUDCBusVolt : Inport
  Data Type Conversion : DataTypeConversion  OutDataTypeStr=uint16  RndMeth=Round  SaturateOnIntegerOverflow=off
  convert_out : FVT_lib/hal/convert_out  gain=0.1  offset=0
  CAN3_Rr_MCUDCBusVolt : Outport
  wires:
  Data Type Conversion/1 -> CAN3_Rr_MCUDCBusVolt/1
  convert_out/1 -> Data Type Conversion/1
  RrMCUDCBusVolt/1 -> convert_out/1

== system halout/HAL_OUT/CAN3/MCU_B_R1_0x190/RrMCUDischrgSta ==
  RrMCUDischrgSta : Inport
  Data Type Conversion : DataTypeConversion  OutDataTypeStr=uint8  RndMeth=Round  SaturateOnIntegerOverflow=off
  CAN3_Rr_MCUDischrgSta : Outport
  wires:
  Data Type Conversion/1 -> CAN3_Rr_MCUDischrgSta/1
  RrMCUDischrgSta/1 -> Data Type Conversion/1

== system halout/HAL_OUT/CAN3/MCU_B_R1_0x190/RrMCUEnaSta ==
  RrMCUEnaSta : Inport
  Data Type Conversion : DataTypeConversion  OutDataTypeStr=uint8  RndMeth=Round  SaturateOnIntegerOverflow=off
  CAN3_Rr_MCUEnaSta : Outport
  wires:
  Data Type Conversion/1 -> CAN3_Rr_MCUEnaSta/1
  RrMCUEnaSta/1 -> Data Type Conversion/1

== system halout/HAL_OUT/CAN3/MCU_B_R1_0x190/RrMCUErr ==
  RrMCUErr : Inport
  Data Type Conversion : DataTypeConversion  OutDataTypeStr=uint8  RndMeth=Round  SaturateOnIntegerOverflow=off
  CAN3_Rr_MCUErr : Outport
  wires:
  Data Type Conversion/1 -> CAN3_Rr_MCUErr/1
  RrMCUErr/1 -> Data Type Conversion/1

== system halout/HAL_OUT/CAN3/MCU_B_R1_0x190/RrMCUIGNsta ==
  RrMCUIGNsta : Inport
  Data Type Conversion : DataTypeConversion  OutDataTypeStr=uint8  RndMeth=Round  SaturateOnIntegerOverflow=off
  CAN3_Rr_MCUIGN_sta : Outport
  wires:
  Data Type Conversion/1 -> CAN3_Rr_MCUIGN_sta/1
  RrMCUIGNsta/1 -> Data Type Conversion/1

== system halout/HAL_OUT/CAN3/MCU_B_R1_0x190/RrMCUReady ==
  RrMCUReady : Inport
  Data Type Conversion : DataTypeConversion  OutDataTypeStr=uint8  RndMeth=Round  SaturateOnIntegerOverflow=off
  CAN3_Rr_MCUReady : Outport
  wires:
  Data Type Conversion/1 -> CAN3_Rr_MCUReady/1
  RrMCUReady/1 -> Data Type Conversion/1

== system halout/HAL_OUT/CAN3/MCU_B_R1_0x190/RrMCUReady4Pre ==
  RrMCUReady4Pre : Inport
  Data Type Conversion : DataTypeConversion  OutDataTypeStr=uint8  RndMeth=Round  SaturateOnIntegerOverflow=off
  CAN3_Rr_MCUReady4Pre : Outport
  wires:
  Data Type Conversion/1 -> CAN3_Rr_MCUReady4Pre/1
  RrMCUReady4Pre/1 -> Data Type Conversion/1

== system halout/HAL_OUT/CAN3/MCU_B_R1_0x190/RrMCUSysSta ==
  RrMCUSysSta : Inport
  Data Type Conversion : DataTypeConversion  OutDataTypeStr=uint8  RndMeth=Round  SaturateOnIntegerOverflow=off
  CAN3_Rr_MCUSysSta : Outport
  wires:
  Data Type Conversion/1 -> CAN3_Rr_MCUSysSta/1
  RrMCUSysSta/1 -> Data Type Conversion/1

== system halout/HAL_OUT/CAN3/MCU_B_R1_0x190/RrMCUTemp ==
  RrMCUTemp : Inport
  Data Type Conversion : DataTypeConversion  OutDataTypeStr=uint16  RndMeth=Round  SaturateOnIntegerOverflow=off
  convert_out : FVT_lib/hal/convert_out  gain=1  offset=-40
  CAN3_Rr_MCUTemp : Outport
  wires:
  Data Type Conversion/1 -> CAN3_Rr_MCUTemp/1
  convert_out/1 -> Data Type Conversion/1
  RrMCUTemp/1 -> convert_out/1

== system halout/HAL_OUT/CAN3/MCU_B_R1_0x190/RrMotorAvailTq ==
  RrMotorAvailTq : Inport
  Data Type Conversion : DataTypeConversion  OutDataTypeStr=uint16  RndMeth=Round  SaturateOnIntegerOverflow=off
  CAN3_Rr_MotorAvailTq : Outport
  wires:
  Data Type Conversion/1 -> CAN3_Rr_MotorAvailTq/1
  RrMotorAvailTq/1 -> Data Type Conversion/1

== system halout/HAL_OUT/CAN3/MCU_B_R1_0x190/RrRegenAvailTq ==
  RrRegenAvailTq : Inport
  Data Type Conversion : DataTypeConversion  OutDataTypeStr=uint16  RndMeth=Round  SaturateOnIntegerOverflow=off
  convert_out : FVT_lib/hal/convert_out  gain=1  offset=-1022
  CAN3_Rr_RegenAvailTq : Outport
  wires:
  Data Type Conversion/1 -> CAN3_Rr_RegenAvailTq/1
  convert_out/1 -> Data Type Conversion/1
  RrRegenAvailTq/1 -> convert_out/1

== system halout/HAL_OUT/CAN3/MCU_B_R1_0x190/RrReservedbits ==
  RrReservedbits : Inport
  Data Type Conversion : DataTypeConversion  OutDataTypeStr=uint8  RndMeth=Round  SaturateOnIntegerOverflow=off
  CAN3_Rr_Reserved_bits : Outport
  wires:
  Data Type Conversion/1 -> CAN3_Rr_Reserved_bits/1
  RrReservedbits/1 -> Data Type Conversion/1

== system halout/HAL_OUT/CAN3/MCU_B_R1_0x190/RrTMSpd ==
  RrTMSpd : Inport
  Data Type Conversion : DataTypeConversion  OutDataTypeStr=uint16  RndMeth=Round  SaturateOnIntegerOverflow=off
  convert_out : FVT_lib/hal/convert_out  gain=1  offset=-18000
  CAN3_Rr_TMSpd : Outport
  wires:
  Data Type Conversion/1 -> CAN3_Rr_TMSpd/1
  convert_out/1 -> Data Type Conversion/1
  RrTMSpd/1 -> convert_out/1

== system halout/HAL_OUT/CAN3/MCU_B_R1_0x190/RrTMTemp ==
  RrTMTemp : Inport
  Data Type Conversion : DataTypeConversion  OutDataTypeStr=uint16  RndMeth=Round  SaturateOnIntegerOverflow=off
  convert_out : FVT_lib/hal/convert_out  gain=1  offset=-40
  CAN3_Rr_TMTemp : Outport
  wires:
  Data Type Conversion/1 -> CAN3_Rr_TMTemp/1
  convert_out/1 -> Data Type Conversion/1
  RrTMTemp/1 -> convert_out/1

== system halout/HAL_OUT/CAN3/MCU_B_R1_0x190/RrTMid ==
  RrTMid : Inport
  Data Type Conversion : DataTypeConversion  OutDataTypeStr=uint16  RndMeth=Round  SaturateOnIntegerOverflow=off
  convert_out : FVT_lib/hal/convert_out  gain=0.1  offset=-1500
  CAN3_Rr_TMid : Outport
  wires:
  Data Type Conversion/1 -> CAN3_Rr_TMid/1
  convert_out/1 -> Data Type Conversion/1
  RrTMid/1 -> convert_out/1

== system halout/HAL_OUT/CAN3/MCU_B_R1_0x190/RrTMiq ==
  RrTMiq : Inport
  Data Type Conversion : DataTypeConversion  OutDataTypeStr=uint16  RndMeth=Round  SaturateOnIntegerOverflow=off
  convert_out : FVT_lib/hal/convert_out  gain=0.1  offset=-1500
  CAN3_Rr_TMiq : Outport
  wires:
  Data Type Conversion/1 -> CAN3_Rr_TMiq/1
  convert_out/1 -> Data Type Conversion/1
  RrTMiq/1 -> convert_out/1

== system halout/HAL_OUT/CAN3/MCU_B_R2_0x193/MCUBRFailLvSta ==
  MCUBRFailLvSta : Inport
  Data Type Conversion : DataTypeConversion  OutDataTypeStr=uint8  RndMeth=Round  SaturateOnIntegerOverflow=off
  CAN3_MCU_B_R_FailLv_Sta : Outport
  wires:
  Data Type Conversion/1 -> CAN3_MCU_B_R_FailLv_Sta/1
  MCUBRFailLvSta/1 -> Data Type Conversion/1

== system halout/HAL_OUT/CAN3/MCU_B_R2_0x193/MCUBRKL302TqCntSta ==
  MCUBRKL302TqCntSta : Inport
  Data Type Conversion : DataTypeConversion  OutDataTypeStr=uint8  RndMeth=Round  SaturateOnIntegerOverflow=off
  CAN3_MCU_B_R_KL302TqCnt_Sta : Outport
  wires:
  Data Type Conversion/1 -> CAN3_MCU_B_R_KL302TqCnt_Sta/1
  MCUBRKL302TqCntSta/1 -> Data Type Conversion/1

== system halout/HAL_OUT/CAN3/MCU_B_R2_0x193/MCUBRLLCTempWarnSta ==
  MCUBRLLCTempWarnSta : Inport
  Data Type Conversion : DataTypeConversion  OutDataTypeStr=uint8  RndMeth=Round  SaturateOnIntegerOverflow=off
  CAN3_MCU_B_R_LLCTempWarn_Sta : Outport
  wires:
  Data Type Conversion/1 -> CAN3_MCU_B_R_LLCTempWarn_Sta/1
  MCUBRLLCTempWarnSta/1 -> Data Type Conversion/1

== system halout/HAL_OUT/CAN3/MCU_B_R2_0x193/RrCoolanttempReq ==
  RrCoolanttempReq : Inport
  Data Type Conversion : DataTypeConversion  OutDataTypeStr=uint16  RndMeth=Round  SaturateOnIntegerOverflow=off
  convert_out : FVT_lib/hal/convert_out  gain=1  offset=-40
  CAN3_Rr_CoolanttempReq : Outport
  wires:
  Data Type Conversion/1 -> CAN3_Rr_CoolanttempReq/1
  convert_out/1 -> Data Type Conversion/1
  RrCoolanttempReq/1 -> convert_out/1

== system halout/HAL_OUT/CAN3/MCU_B_R2_0x193/RrFailcode1 ==
  RrFailcode1 : Inport
  Data Type Conversion : DataTypeConversion  OutDataTypeStr=uint8  RndMeth=Round  SaturateOnIntegerOverflow=off
  CAN3_Rr_Failcode1 : Outport
  wires:
  Data Type Conversion/1 -> CAN3_Rr_Failcode1/1
  RrFailcode1/1 -> Data Type Conversion/1

== system halout/HAL_OUT/CAN3/MCU_B_R2_0x193/RrFailcode2 ==
  RrFailcode2 : Inport
  Data Type Conversion : DataTypeConversion  OutDataTypeStr=uint8  RndMeth=Round  SaturateOnIntegerOverflow=off
  CAN3_Rr_Failcode2 : Outport
  wires:
  Data Type Conversion/1 -> CAN3_Rr_Failcode2/1
  RrFailcode2/1 -> Data Type Conversion/1

== system halout/HAL_OUT/CAN3/MCU_B_R2_0x193/RrFailcodehistory1 ==
  RrFailcodehistory1 : Inport
  Data Type Conversion : DataTypeConversion  OutDataTypeStr=uint8  RndMeth=Round  SaturateOnIntegerOverflow=off
  CAN3_Rr_Failcodehistory1 : Outport
  wires:
  Data Type Conversion/1 -> CAN3_Rr_Failcodehistory1/1
  RrFailcodehistory1/1 -> Data Type Conversion/1

== system halout/HAL_OUT/CAN3/MCU_B_R2_0x193/RrFailcodehistory2 ==
  RrFailcodehistory2 : Inport
  Data Type Conversion : DataTypeConversion  OutDataTypeStr=uint8  RndMeth=Round  SaturateOnIntegerOverflow=off
  CAN3_Rr_Failcodehistory2 : Outport
  wires:
  Data Type Conversion/1 -> CAN3_Rr_Failcodehistory2/1
  RrFailcodehistory2/1 -> Data Type Conversion/1

== system halout/HAL_OUT/CAN3/MCU_B_R2_0x193/RrLLCTemp ==
  RrLLCTemp : Inport
  Data Type Conversion : DataTypeConversion  OutDataTypeStr=uint16  RndMeth=Round  SaturateOnIntegerOverflow=off
  convert_out : FVT_lib/hal/convert_out  gain=1  offset=-40
  CAN3_Rr_LLCTemp : Outport
  wires:
  Data Type Conversion/1 -> CAN3_Rr_LLCTemp/1
  convert_out/1 -> Data Type Conversion/1
  RrLLCTemp/1 -> convert_out/1

== system halout/HAL_OUT/CAN3/MCU_B_R2_0x193/RrLLCflowReq ==
  RrLLCflowReq : Inport
  Data Type Conversion : DataTypeConversion  OutDataTypeStr=uint8  RndMeth=Round  SaturateOnIntegerOverflow=off
  convert_out : FVT_lib/hal/convert_out  gain=0.25  offset=0
  CAN3_Rr_LLCflowReq : Outport
  wires:
  Data Type Conversion/1 -> CAN3_Rr_LLCflowReq/1
  convert_out/1 -> Data Type Conversion/1
  RrLLCflowReq/1 -> convert_out/1

== system halout/HAL_OUT/CAN3/MCU_B_R2_0x193/RrMCU2Chksum ==
  RrMCU2Chksum : Inport
  Data Type Conversion : DataTypeConversion  OutDataTypeStr=uint8  RndMeth=Round  SaturateOnIntegerOverflow=off
  CAN3_Rr_MCU2Chksum : Outport
  wires:
  Data Type Conversion/1 -> CAN3_Rr_MCU2Chksum/1
  RrMCU2Chksum/1 -> Data Type Conversion/1

== system halout/HAL_OUT/CAN3/MCU_B_R2_0x193/RrMCU2RolCnt ==
  RrMCU2RolCnt : Inport
  Data Type Conversion : DataTypeConversion  OutDataTypeStr=uint8  RndMeth=Round  SaturateOnIntegerOverflow=off
  CAN3_Rr_MCU2RolCnt : Outport
  wires:
  Data Type Conversion/1 -> CAN3_Rr_MCU2RolCnt/1
  RrMCU2RolCnt/1 -> Data Type Conversion/1

== system halout/HAL_OUT/CAN3/MCU_B_R2_0x193/RrMCU3HWVer ==
  RrMCU3HWVer : Inport
  Data Type Conversion : DataTypeConversion  OutDataTypeStr=uint16  RndMeth=Round  SaturateOnIntegerOverflow=off
  CAN3_Rr_MCU3_HW_Ver : Outport
  wires:
  Data Type Conversion/1 -> CAN3_Rr_MCU3_HW_Ver/1
  RrMCU3HWVer/1 -> Data Type Conversion/1

== system halout/HAL_OUT/CAN3/MCU_B_R2_0x193/RrMCU3SWVer ==
  RrMCU3SWVer : Inport
  Data Type Conversion : DataTypeConversion  OutDataTypeStr=uint16  RndMeth=Round  SaturateOnIntegerOverflow=off
  CAN3_Rr_MCU3_SW_Ver : Outport
  wires:
  Data Type Conversion/1 -> CAN3_Rr_MCU3_SW_Ver/1
  RrMCU3SWVer/1 -> Data Type Conversion/1

== system halout/HAL_OUT/CAN3/MCU_B_R2_0x193/RrMCUTempWarn ==
  RrMCUTempWarn : Inport
  Data Type Conversion : DataTypeConversion  OutDataTypeStr=uint8  RndMeth=Round  SaturateOnIntegerOverflow=off
  CAN3_Rr_MCUTempWarn : Outport
  wires:
  Data Type Conversion/1 -> CAN3_Rr_MCUTempWarn/1
  RrMCUTempWarn/1 -> Data Type Conversion/1

== system halout/HAL_OUT/CAN3/MCU_B_R2_0x193/RrTMTempWarn ==
  RrTMTempWarn : Inport
  Data Type Conversion : DataTypeConversion  OutDataTypeStr=uint8  RndMeth=Round  SaturateOnIntegerOverflow=off
  CAN3_Rr_TMTempWarn : Outport
  wires:
  Data Type Conversion/1 -> CAN3_Rr_TMTempWarn/1
  RrTMTempWarn/1 -> Data Type Conversion/1

== system halout/HAL_OUT/CAN3/MCU_FVT_R1_0x199/MCUFVTRBoostOPSta ==
  MCUFVTRBoostOPSta : Inport
  Data Type Conversion : DataTypeConversion  OutDataTypeStr=uint8  RndMeth=Round  SaturateOnIntegerOverflow=off
  CAN3_MCU_FVT_R_BoostOP_Sta : Outport
  wires:
  Data Type Conversion/1 -> CAN3_MCU_FVT_R_BoostOP_Sta/1
  MCUFVTRBoostOPSta/1 -> Data Type Conversion/1

== system halout/HAL_OUT/CAN3/MCU_FVT_R1_0x199/MCUFVTREDUTqReqFbk ==
  MCUFVTREDUTqReqFbk : Inport
  Data Type Conversion : DataTypeConversion  OutDataTypeStr=uint16  RndMeth=Round  SaturateOnIntegerOverflow=off
  convert_out : FVT_lib/hal/convert_out  gain=0.1  offset=-1022
  CAN3_MCU_FVT_R_EDUTqReq_Fbk : Outport
  wires:
  Data Type Conversion/1 -> CAN3_MCU_FVT_R_EDUTqReq_Fbk/1
  convert_out/1 -> Data Type Conversion/1
  MCUFVTREDUTqReqFbk/1 -> convert_out/1

== system halout/HAL_OUT/CAN3/MCU_FVT_R1_0x199/MCUFVTRFailcode3Sta ==
  MCUFVTRFailcode3Sta : Inport
  Data Type Conversion : DataTypeConversion  OutDataTypeStr=uint8  RndMeth=Round  SaturateOnIntegerOverflow=off
  CAN3_MCU_FVT_R_Failcode3_Sta : Outport
  wires:
  Data Type Conversion/1 -> CAN3_MCU_FVT_R_Failcode3_Sta/1
  MCUFVTRFailcode3Sta/1 -> Data Type Conversion/1

== system halout/HAL_OUT/CAN3/MCU_FVT_R1_0x199/MCUFVTRHeatingOPSta ==
  MCUFVTRHeatingOPSta : Inport
  Data Type Conversion : DataTypeConversion  OutDataTypeStr=uint8  RndMeth=Round  SaturateOnIntegerOverflow=off
  CAN3_MCU_FVT_R_HeatingOP_Sta : Outport
  wires:
  Data Type Conversion/1 -> CAN3_MCU_FVT_R_HeatingOP_Sta/1
  MCUFVTRHeatingOPSta/1 -> Data Type Conversion/1

== system halout/HAL_OUT/CAN3/MCU_FVT_R1_0x199/MCUFVTRMCUBATSta ==
  MCUFVTRMCUBATSta : Inport
  Data Type Conversion : DataTypeConversion  OutDataTypeStr=uint16  RndMeth=Round  SaturateOnIntegerOverflow=off
  convert_out : FVT_lib/hal/convert_out  gain=0.2  offset=0
  CAN3_MCU_FVT_R_MCUBAT_Sta : Outport
  wires:
  Data Type Conversion/1 -> CAN3_MCU_FVT_R_MCUBAT_Sta/1
  convert_out/1 -> Data Type Conversion/1
  MCUFVTRMCUBATSta/1 -> convert_out/1

== system halout/HAL_OUT/CAN3/MCU_FVT_R1_0x199/MCUFVTRMCUErrSta ==
  MCUFVTRMCUErrSta : Inport
  Data Type Conversion : DataTypeConversion  OutDataTypeStr=uint8  RndMeth=Round  SaturateOnIntegerOverflow=off
  CAN3_MCU_FVT_R_MCUErr_Sta : Outport
  wires:
  Data Type Conversion/1 -> CAN3_MCU_FVT_R_MCUErr_Sta/1
  MCUFVTRMCUErrSta/1 -> Data Type Conversion/1

== system halout/HAL_OUT/CAN3/MCU_FVT_R1_0x199/MCUFVTRMCUSysSta ==
  MCUFVTRMCUSysSta : Inport
  Data Type Conversion : DataTypeConversion  OutDataTypeStr=uint8  RndMeth=Round  SaturateOnIntegerOverflow=off
  CAN3_MCU_FVT_R_MCUSys_Sta : Outport
  wires:
  Data Type Conversion/1 -> CAN3_MCU_FVT_R_MCUSys_Sta/1
  MCUFVTRMCUSysSta/1 -> Data Type Conversion/1

== system halout/HAL_OUT/CAN3/MCU_FVT_R1_0x199/MCUFVTROilTempSta ==
  MCUFVTROilTempSta : Inport
  Data Type Conversion : DataTypeConversion  OutDataTypeStr=uint16  RndMeth=Round  SaturateOnIntegerOverflow=off
  convert_out : FVT_lib/hal/convert_out  gain=1  offset=-40
  CAN3_MCU_FVT_R_OilTemp_Sta : Outport
  wires:
  Data Type Conversion/1 -> CAN3_MCU_FVT_R_OilTemp_Sta/1
  convert_out/1 -> Data Type Conversion/1
  MCUFVTROilTempSta/1 -> convert_out/1

== system halout/HAL_OUT/CAN3/MCU_FVT_R1_0x199/MCUFVTRTMSpdSta ==
  MCUFVTRTMSpdSta : Inport
  Data Type Conversion : DataTypeConversion  OutDataTypeStr=uint16  RndMeth=Round  SaturateOnIntegerOverflow=off
  convert_out : FVT_lib/hal/convert_out  gain=1  offset=-22000
  CAN3_MCU_FVT_R_TMSpd_Sta : Outport
  wires:
  Data Type Conversion/1 -> CAN3_MCU_FVT_R_TMSpd_Sta/1
  convert_out/1 -> Data Type Conversion/1
  MCUFVTRTMSpdSta/1 -> convert_out/1

== system halout/HAL_OUT/CAN_MCU_R1/MCU_FVT_R_Local1_0x3F0/MCUFVTRLocal1CSSta ==
  MCUFVTRLocal1CSSta : Inport
  Data Type Conversion : DataTypeConversion  OutDataTypeStr=uint8  RndMeth=Round  SaturateOnIntegerOverflow=off
  CAN_MCU_R1_MCU_FVT_R_Local1_CS_Sta : Outport
  wires:
  Data Type Conversion/1 -> CAN_MCU_R1_MCU_FVT_R_Local1_CS_Sta/1
  MCUFVTRLocal1CSSta/1 -> Data Type Conversion/1

== system halout/HAL_OUT/CAN_MCU_R1/MCU_FVT_R_Local1_0x3F0/MCUFVTRLocal1RCSta ==
  MCUFVTRLocal1RCSta : Inport
  Data Type Conversion : DataTypeConversion  OutDataTypeStr=uint8  RndMeth=Round  SaturateOnIntegerOverflow=off
  CAN_MCU_R1_MCU_FVT_R_Local1_RC_Sta : Outport
  wires:
  Data Type Conversion/1 -> CAN_MCU_R1_MCU_FVT_R_Local1_RC_Sta/1
  MCUFVTRLocal1RCSta/1 -> Data Type Conversion/1

== system halout/HAL_OUT/CAN_MCU_R1/MCU_FVT_R_Local1_0x3F0/MCUFVTROPCStartOnReq ==
  MCUFVTROPCStartOnReq : Inport
  Data Type Conversion : DataTypeConversion  OutDataTypeStr=uint8  RndMeth=Round  SaturateOnIntegerOverflow=off
  CAN_MCU_R1_MCU_FVT_R_OPCStartOn_Req : Outport
  wires:
  Data Type Conversion/1 -> CAN_MCU_R1_MCU_FVT_R_OPCStartOn_Req/1
  MCUFVTROPCStartOnReq/1 -> Data Type Conversion/1

== system halout/HAL_OUT/CAN_MCU_R1/MCU_FVT_R_Local1_0x3F0/MCUFVTROilPmpTarSpdReq ==
  MCUFVTROilPmpTarSpdReq : Inport
  Data Type Conversion : DataTypeConversion  OutDataTypeStr=uint16  RndMeth=Round  SaturateOnIntegerOverflow=off
  CAN_MCU_R1_MCU_FVT_R_OilPmpTarSpd_Req : Outport
  wires:
  Data Type Conversion/1 -> CAN_MCU_R1_MCU_FVT_R_OilPmpTarSpd_Req/1
  MCUFVTROilPmpTarSpdReq/1 -> Data Type Conversion/1

== stateflow chart halout/HAL_OUT/CAN_Scheduler ==
  state CAN_scheduler
    (default) -> (junction 55)
    CAN_scheduler -> (junction 55)
    (junction 55) -> (junction 53) [order 1] : [KHAL_CAN_MCU_R1TxReq_flg && VOUTP_ALLCANTxReq_flg]
    (junction 55) -> (junction 214) [order 2]
    (junction 53) -> (junction 212) : {
        | trig_can_mcu_r1;
        | }
    (junction 212) -> (junction 214)
    (junction 214) -> (junction 250)
    (junction 250) -> (junction 251) [order 1] : [KHAL_CAN3TxReq_flg && VOUTP_ALLCANTxReq_flg]
    (junction 250) -> (junction 253) [order 2]
    (junction 251) -> (junction 247) : {
        | trig_can3;
        | }
    (junction 247) -> (junction 253)
  data: KHAL_CAN3TxReq_flg input; VOUTP_ALLCANTxReq_flg input; KHAL_CAN_MCU_R1TxReq_flg input
  events: trig_can_mcu_r1 output FUNCTION_CALL_EVENT; trig_can3 output FUNCTION_CALL_EVENT
